simulink model "Expt_5_1"  (R2018a)
settings: Solver=VariableStepAuto  StartTime=0.0  StopTime=10.0  RelTol=1e-3
libraries: simulink x1
settings Model: Creator=HP  LastModifiedBy=HP

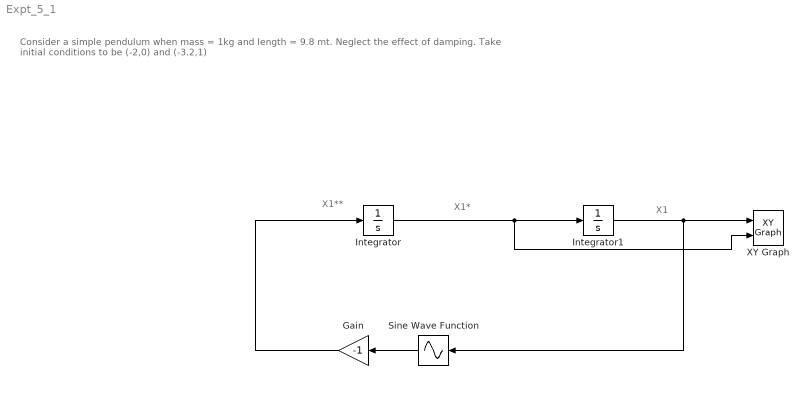
== system Expt_5_1 ==
  note: X1
  note: X1*
  note: X1**
  note: Consider a simple pendulum when mass = 1kg and length = 9.8 mt.
      | Neglect the effect of damping.
      | Take initial conditions to be (-2,0) and (-3.2,1)
  Gain : Gain  Gain=-1
  Integrator : Integrator  InitialCondition=1
  Integrator1 : Integrator  InitialCondition=-3.2
  Sine Wave Function : Sin  TimeSource=Use external signal  SampleTime=0
  XY Graph : simulink/Sinks/XY Graph  xmin=-10  xmax=10  ymin=-10  ymax=10  st=-1
  wires:
  Integrator1/1 -> Sine Wave Function/1, XY Graph/1
  Integrator/1 -> XY Graph/2, Integrator1/1
  Sine Wave Function/1 -> Gain/1
  Gain/1 -> Integrator/1
